simulink model "simulink_inverse_kinematics"  (R2025b)
settings: Solver=VariableStepAuto  StartTime=0.0  StopTime=1  RelTol=1e-3
undefined symbols (not defined in the file): EE_target_DCM, EE_target_POS, home_configuration, Levenberg, Marquardt, weight
libraries: robotcorelib x1, robotmaniplib x1
settings Model: Creator=matte  LastModifiedBy=mdambrosio

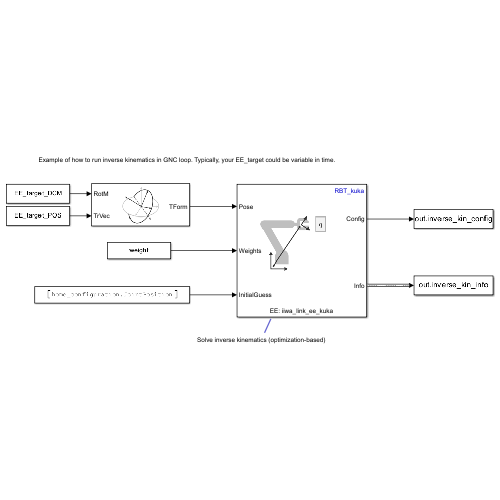
[thumbnail: Simulink's stored preview of the top-level diagram]
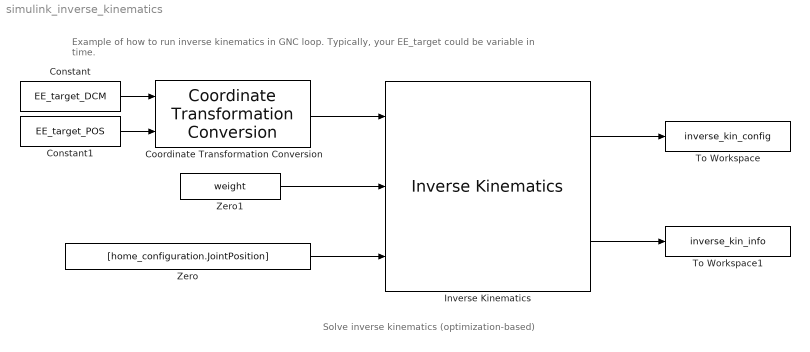
== system simulink_inverse_kinematics ==
  note: Example of how to run inverse kinematics in GNC loop. Typically, your EE_target could be variable in time.
  note: Solve inverse kinematics (optimization-based)
  Constant : Constant  Value=EE_target_DCM
  Constant1 : Constant  Value=EE_target_POS
  Coordinate Transformation Conversion : robotcorelib/Coordinate Transformation Conversion  InputRepresentation=Rotation Matrix  InputEulerSequence=ZYX  ShowTrVecInputPort=on  OutputRepresentation=Homogeneous Transformation  OutputEulerSequence=ZYX  ShowTrVecOutputPort=on  SimulateUsing=Interpreted execution
      settings: LibrarySourceBlock=navlib/Utilities/Coordinate Transformation Conversion
  Inverse Kinematics : robotmaniplib/Inverse Kinematics  RigidBodyTree=RBT_kuka  EndEffector=iiwa_link_ee_kuka  ShowInfo=on  SolverName=Levenberg-Marquardt  EnforceJointLimits=on  MaxIterations=1500  MaxTime=10  GradientTolerance=1e-7  SolutionTolerance=1e-6  StepTolerance=1e-14  ConstraintTolerance=1e-6  ErrorChangeTolerance=1e-12  UseErrorDamping=on  DampingBias=0.0025  SimulateUsing=Interpreted execution
  To Workspace : ToWorkspace  VariableName=inverse_kin_config  SaveFormat=Structure  SampleTime=-1
  To Workspace1 : ToWorkspace  VariableName=inverse_kin_info  SaveFormat=Timeseries  SampleTime=-1
  Zero : Constant  Value=[home_configuration.JointPosition]  OutDataTypeStr=Inherit: Inherit via back propagation
  Zero1 : Constant  Value=weight  OutDataTypeStr=Inherit: Inherit via back propagation
  wires:
  Zero/1 -> Inverse Kinematics/3
  Zero1/1 -> Inverse Kinematics/2
  Constant/1 -> Coordinate Transformation Conversion/1
  Constant1/1 -> Coordinate Transformation Conversion/2
  Coordinate Transformation Conversion/1 -> Inverse Kinematics/1
  Inverse Kinematics/1 -> To Workspace/1
  Inverse Kinematics/2 -> To Workspace1/1
